simulink model "DR18E_Testpult"  (R2017a)
settings: Solver=ode1  StartTime=0.0  StopTime=Inf  FixedStep=0.001  RelTol=1e-3
PostLoadFcn:
  | , if any(exist('dsrtsu_mdlpostloadfcn', 'file') == [2, 3, 6]), try dsrtsu_mdlpostloadfcn('Execute', bdroot); catch fprintf('Error in PostLoadFcn (dsrtsu_mdlpostloadfcn) for model "%s":\n %s\n', bdroot, lasterr); end, end,
model workspace: external: MATLAB File C:\Users\DeltaRacing\Documents\dSPACE\MABX_DR18E\Model\DR18E_MABX_Parameter.m (data not in the file)
values from neighbouring files (symbols this model uses):
  am = 1/Ts    (= 1)    [DR18E_MABX_Parameter.m]
  bm = K/Ts    (= 0.05)    [DR18E_MABX_Parameter.m]
  cf = 41350    [DR18E_MABX_Parameter.m]
  cr = 41350    [DR18E_MABX_Parameter.m]
  Derating_HV_Battery_Kapa = 1    [DR18E_MABX_Parameter.m]
  Derating_Start_km = 16    [DR18E_MABX_Parameter.m]
  Drive_Mode = 0    [DR18E_MABX_Parameter.m]
  g = 1    [DR18E_MABX_Parameter.m]
  Gas_Modus = 2    [DR18E_MABX_Parameter.m]
  HV_Power_max = 80    [DR18E_MABX_Parameter.m]
  i_Getriebe = 3.3    [DR18E_MABX_Parameter.m]
  i_Lenkgetriebe = 4.32    [DR18E_MABX_Parameter.m]
  K_SET = 1    [DR18E_MABX_Parameter.m]
  Kapazitaet_HV_Battery_kWh = 6.6    [DR18E_MABX_Parameter.m]
  KW_T_Soll = 37    [DR18E_MABX_Parameter.m]
  lf = 1.2    [DR18E_MABX_Parameter.m]
  lr = 1.15    [DR18E_MABX_Parameter.m]
  m = 310    [DR18E_MABX_Parameter.m]
  M_max = 150    [DR18E_MABX_Parameter.m]
  Power_Limit_onoff = 0    [DR18E_MABX_Parameter.m]
  Reifenradius = 0.2351    [DR18E_MABX_Parameter.m]
  Strecke_Endu_km = 22    [DR18E_MABX_Parameter.m]
  TC_Decr_Gas = 0.00005    (= 5e-05)    [DR18E_MABX_Parameter.m]
  TC_Derivative = 0.4    [DR18E_MABX_Parameter.m]
  TC_Incr_Gas = 0.005    [DR18E_MABX_Parameter.m]
  TC_On = 0    [DR18E_MABX_Parameter.m]
  TC_Relay_Off = 0.065    [DR18E_MABX_Parameter.m]
  TC_Relay_On = 0.07    [DR18E_MABX_Parameter.m]
  TV_Mode = 2    [DR18E_MABX_Parameter.m]
  TV_On = 0    [DR18E_MABX_Parameter.m]
  TV_Override = 1    [DR18E_MABX_Parameter.m]
  y = 0.8    [DR18E_MABX_Parameter.m]
undefined symbols (not defined in the file or in its folder): D, DiscIntNeverNeededParam, I, K_OL, P
libraries: simulink x288, rtican x105, rtiusbflightreclib x40, rti1401lib_dio_type3 x10, simulink_extras x10, rti1401lib_adc_type4 x8, rti1401lib_II_base x7
(part 1 of 28)
Description:
  | Standard RTI1401 template.
  | Supported Matlab version:  R2017a.
settings Model: Tag=RTI1401  DSRTSU_INTERNAL_RTI_VER=500  DSRTSU_INTERNAL_RTI_TYPE=rti1401  DSRTSU_INTERNAL_RTIFPGA=90  Creator=DeltaRacing  LastModifiedBy=DeltaRacing
settings OptimizationCC: BlockReduction=off  OptimizeBlockIOStorage=off  BufferReuse=off  GlobalBufferReuse=off  ExpressionFolding=off  LocalBlockOutputs=off
settings DebuggingCC: SFNoUnconditionalDefaultTransitionDiag=warning
settings HardwareCC: ProdBitPerPointer=32  ProdBitPerSizeT=32  ProdBitPerPtrDiffT=32  ProdLargestAtomicInteger=Integer  ProdEndianess=BigEndian  ProdWordSize=32  ProdHWDeviceType=Custom Processor->Custom  TargetIntDivRoundTo=Zero  TargetEndianess=BigEndian  TargetHWDeviceType=Custom Processor->Custom
settings SFSimCC: MATLABDynamicMemAlloc=off
settings RTWCC: SystemTargetFile=rti1401.tlc  MakeCommand=make_rti  TemplateMakefile=rti1401.tmf  Description=dSPACE DS1401 Hardware Platform
settings RTWCC: CustomSource=|
  | flightrecsetup.c
  | DsFlRecUSB.c
settings STFCustomTargetCC: ParMdlRefBuildCompliant=on  GRTInterface=off  SystemTargetFile=rti1401.tlc
settings GRTTargetCC: TargetLangStandard=C89/C90 (ANSI)  CompOptLevelCompliant=off  ConcurrentExecutionCompliant=off  CombineOutputUpdateFcns=off  MatFileLogging=off  CPPClassGenCompliant=off  UseToolchainInfoCompliant=off
settings ConfigComp: CovMetricSettings=dswe

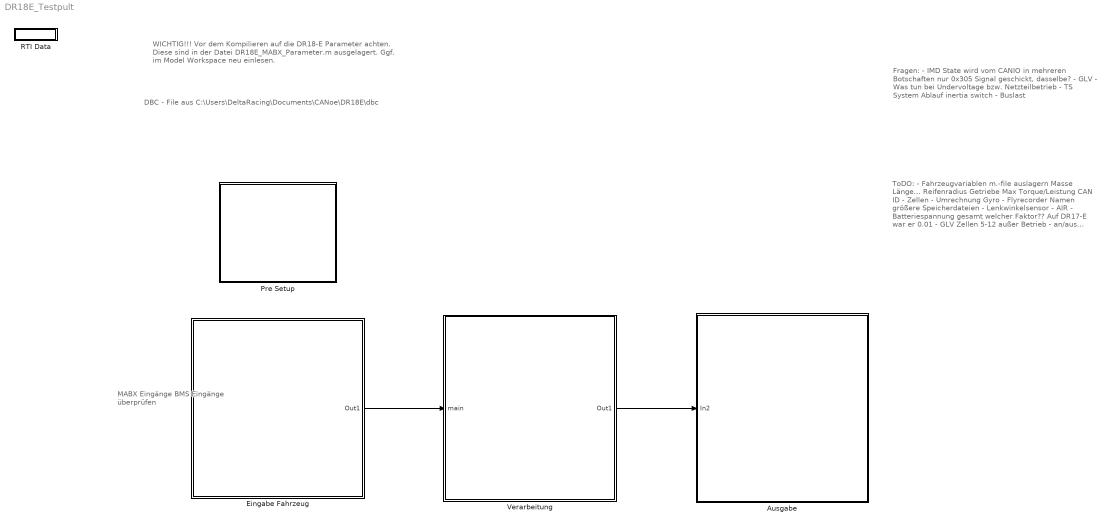
== system DR18E_Testpult ==
  note: WICHTIG!!!
      |
      | Vor dem Kompilieren auf die DR18-E Parameter achten.
      | Diese sind in der Datei DR18E_MABX_Parameter.m ausgelagert.
      | Ggf. im Model Workspace neu einlesen.
  note: MABX Eingänge
      | BMS Eingänge
      |
      | überprüfen
  note: DBC - File aus C:\Users\DeltaRacing\Documents\CANoe\DR18E\dbc
  note: Fragen:
      |
      | - IMD State wird vom CANIO in mehreren Botschaften
      | 		nur 0x305 Signal
      |  geschickt, dasselbe?
      | - GLV - Was tun bei Undervoltage bzw. Netzteilbetrieb
      | - TS System Ablauf
      | 	inertia switch
      | - Buslast
  note: ToDO:
      |
      | - Fahrzeugvariablen m.-file auslagern
      | 	Masse
      | 	Länge...
      | 	Reifenradius
      | 	Getriebe
      | 	Max Torque/Leistung
      | 	CAN ID - Zellen
      | - Umrechnung Gyro
      | - Flyrecorder
      | 	Namen
      | 	größere Speicherdateien
      | - Lenkwinkelsensor
      | - AIR
      | - Batteriespannung gesamt
      | 	welcher Faktor?? Auf DR17-E war er 0.01
      | - GLV Zellen 5-12 außer Betrieb
      | - an/aus Signale in dbc verankern (mal 255)
      | 	in dbc unsigned Variable und Faktor 255
      | - Sendezeiten in der dbc üperprüfen
      | 		Botschaft/Signal.. onchange cyclic
      | - TV Torque dazuaddieren Regel raussuchen
      | - BMS Generell
      | 		AMS Relay, 0x170, 0x231-2
      | - Unterschied zw. Speaker und Sound - State Machine
      | - Inverter Status Fehler Bit 31 überprüfen
      | - Skalierung Inverterwerte
      | 	Drehzahl Umrechung - 4000/2^15
      | 	Warum 4000?
      | - Rückwärtsgang
      | - BSPD Status - NOT OPERATOR? Warum
  Ausgabe : Subsystem
  Eingabe Fahrzeug : Subsystem
  Pre Setup : Subsystem
  RTI Data : Subsystem  Tag=struct('RTIDataServer',struct('RTIDataServerVs','2','RTIModelDescription','struct(''main'',''DR18E_Testpult'',''sub'','''',''isMp'',0)'))  LoadFcn="if exist('rtidc'), try,  rtidc('DataHostBlockClbLoad', gcbh); catch, disp(['Warning: ''LoadFcn'' for RTI Data block failed: ' lasterr]); end, end,"  mask(RTI_DATA_HOST){}
      mask help:
      | RTI Data Block.
      | This block is used by RTI to store internal model-dependent data.
      | Please keep this block on the root level of the model. Deleting this block will result in data loss.
      |
      | NEVER DELETE OR COPY THIS BLOCK!
      settings: CopyFcn="if exist('rtidc'), try,  rtidc('DataHostBlockClbCopy', gcbh); catch, disp(['Warning: ''CopyFcn'' for RTI Data block failed: ' lasterr]); end, end,"  DeleteFcn="if exist('rtidc'), try,  rtidc('DataHostBlockClbDelete', gcbh); catch, disp(['Warning: ''DeleteFcn'' for RTI Data block failed: ' lasterr]); end, end,"  ModelCloseFcn="if exist('rtidc'), try,  rtidc('DataHostBlockClbModelClose', gcbh); catch, disp(['Warning: ''ModelCloseFcn'' for RTI Data block failed: ' lasterr]); end, end,"  PreSaveFcn="if exist('rtidc'), try,  rtidc('DataHostBlockClbPreSave', gcbh); catch, disp(['Warning: ''PreSaveFcn'' for RTI Data block failed: ' lasterr]); end, end,"  PostSaveFcn="if exist('rtidc'), try,  rtidc('DataHostBlockClbPostSave', gcbh); catch, disp(['Warning: ''PostSaveFcn'' for RTI Data block failed: ' lasterr]); end, end,"  NameChangeFcn="if exist('rtidc'), try,  rtidc('DataHostBlockClbNameChange', gcbh); catch, disp(['Warning: ''NameChangeFcn'' for RTI Data block failed: ' lasterr]); end, end,"
      mask Help:
      | RTI Data Block.
      | This block is used by RTI to store internal model-dependent data.
      | Please keep this block on the root level of the model. Deleting this block will result in data loss.
      | 
      | NEVER DELETE OR COPY THIS BLOCK!
      mask Display:
      | text(0.5, 0.5, 'RTI Data', 'HorizontalAlignment', 'center');
      | plot([1 0]);
  Verarbeitung : Subsystem
  wires:
  Eingabe Fahrzeug/1(Out1) -> Verarbeitung/1(main)
  Verarbeitung/1(Out1) -> Ausgabe/1(In2)

== system DR18E_Testpult/Ausgabe ==
  In2 : Inport
  AMS : Subsystem
  Bus Selector : BusSelector  OutputSignals=Outputs_StateMachine.O_Inverter_TX_Mode,Outputs_StateMachine.UmrichterInit,Torque_L_R_Nm,Outputs_StateMachine.UniversalTX.RegID_L_R,Outputs_StateMachine.UniversalTX.Value32_L_R
  Bus Selector1 : BusSelector  OutputSignals=Outputs_StateMachine.O_Sicherheitskreis_Enable,Bremse_bin,Outputs_StateMachine.O_SpeakerEnable,PumpePWM,LüfterPWM,Outputs_StateMachine.O_Precharge_Enable,Outputs_StateMachine.O_InverterFRE
  Bus Selector2 : BusSelector  OutputSignals=Outputs_StateMachine.O_ErrorNr,Outputs_StateMachine.O_State,M_max,LED Bar Vektor.LED Bar Vektor
  Bus Selector3 : BusSelector  OutputSignals=Outputs_StateMachine.O_fBlink_Start,Sicherheitskreis,LV_Undervoltage
  Bus Selector4 : BusSelector  OutputSignals=A_AMS_out,A_IMD_out
  Bus Selector5 : BusSelector  OutputSignals=Lüfter HV Battery
  Bus Selector6 : BusSelector  OutputSignals=Bus_Input.Umrichter.U1.Mot_Temp,Bus_Input.Umrichter.U2.Mot_Temp,Bus_Input.Umrichter.U1.InverterTemp,Bus_Input.Umrichter.U2.InverterTemp
  CANIO : Subsystem
  Diagnose : Subsystem
  Display : Subsystem
  Inverter TX : Subsystem
  SensorboardMitte : Subsystem
  or : Logic  Operator=OR  AllPortsSameDT=off  OutDataTypeStr=boolean
  wires:
  In2/1 -> Bus Selector6/1, Bus Selector5/1, Bus Selector1/1, Bus Selector/1, Bus Selector3/1, Bus Selector2/1
  Bus Selector1/1 -> CANIO/1(Sicherheitskreis)  "<O_Sicherheitskreis_Enable>"
  Bus Selector1/3 -> CANIO/3(Speaker)  "<O_SpeakerEnable>"
  Bus Selector1/4 -> CANIO/4(Wasserpumpe)  "<PumpePWM>"
  Bus Selector1/5 -> CANIO/5(Lüfter)  "<LüfterPWM>"
  Bus Selector1/6 -> CANIO/6(Precharge)  "<O_Precharge_Enable>"
  Bus Selector1/7 -> CANIO/7(Inverter Enable)  "<O_InverterFRE>"
  Bus Selector/1 -> Inverter TX/1(Inverter_TX_Mode)  "<O_Inverter_TX_Mode>"
  Bus Selector/2 -> Inverter TX/2(Init_Values)  "<UmrichterInit>"
  Bus Selector/3 -> Inverter TX/3(Torque_L_R_Nm)  "<Torque_L_R_Nm>"
  Bus Selector/4 -> Inverter TX/4(RegID_L_R1)  "<RegID_L_R>"
  Bus Selector/5 -> Inverter TX/5(Values_L_R_32bit)  "<Value32_L_R>"
  Bus Selector2/1 -> Display/1(ErrorNo)  "<O_ErrorNr>"
  Bus Selector2/2 -> Display/2(State)  "<O_State>"
  Bus Selector3/1 -> SensorboardMitte/1(Starttaster)  "<O_fBlink_Start>"
  Bus Selector1/2 -> CANIO/2(Bremslicht)  "<Bremse_bin>"
  Bus Selector3/2 -> SensorboardMitte/2(DasboardNotausLed)  "<Sicherheitskreis>"
  [vec_Sicherheitskreis] -> Bus Selector4/1
  Bus Selector4/2 -> SensorboardMitte/4(DashboardIMDLed)  "<A_IMD_out>"
  Bus Selector3/3 -> or/1  "<LV_Undervoltage>"
  Bus Selector4/1 -> or/2  "<A_AMS_out>"
  or/1 -> SensorboardMitte/3("DashboardAMSLed ")
  Bus Selector5/1 -> AMS/1(Lüfter HV Battery)  "<Lüfter HV Battery>"
  Bus Selector2/3 -> Display/3("TorqueMax ")  "<M_max>"
  Bus Selector2/4 -> Display/4(LED Bar)  "<LED Bar Vektor>"
  Bus Selector6/1 -> Diagnose/1(Motor 1 Temperatur)  "<Mot_Temp>"
  Bus Selector6/2 -> Diagnose/2(Motor 2 Temperatur)  "<Mot_Temp>"
  Bus Selector6/3 -> Diagnose/3(IGBT 1 Temperatur)  "<InverterTemp>"
  Bus Selector6/4 -> Diagnose/4(IGBT 2 Temperatur)  "<InverterTemp>"

== system DR18E_Testpult/Eingabe Fahrzeug ==
  BMS : Subsystem
  Bus Creator : BusCreator  Inputs=11
  CAN IO : Subsystem
  "GLV AMS " : Subsystem
  Gyro : Subsystem
  Inverter Feedback Messages : Subsystem
  Lenkwinkelgeber : Subsystem
  MicroAutoBox : Subsystem
  Sensorboard Front : Subsystem
  Sensorboard Mitte : Subsystem
  Sensorboard Rear : Subsystem
  Out1 : Outport
  wires:
  Bus Creator/1 -> Out1/1
  Gyro/1(Gyro) -> Bus Creator/2
  Sensorboard Mitte/1(SensorboardMitteOut) -> Bus Creator/3
  Sensorboard Front/1(SensorboardFrontOut) -> Bus Creator/1
  MicroAutoBox/1(MicroAutoBox) -> Bus Creator/11
  Lenkwinkelgeber/1(LenkwinkelgeberOut) -> Bus Creator/5
  Inverter Feedback Messages/1(Out1) -> Bus Creator/6
  BMS/1(BMS Voltage) -> Bus Creator/7
  CAN IO/1(CANIOOut) -> Bus Creator/9
  Sensorboard Rear/1(SensorboardRearOut) -> Bus Creator/4
  "GLV AMS "/1(GLVAMSOut) -> Bus Creator/10
  BMS/2(Out2) -> Bus Creator/8

== system DR18E_Testpult/Pre Setup ==
  note: MABX ZIF Connector
      | CAN 3
  note: MABX ZIF Connector
      | CAN 1
  note: MABX ZIF Connector
      | CAN 2
  CAN 1 - Body : rtican/RTICAN CONTROLLER SETUP   Reserved1=[]  Reserved2=[]  Reserved3=[]  Reserved4=[]  AcceptanceMask=[]  ArbitrationField=[]  Parameters=[]  SFcnRTICANSettings=[]  MS_Struct=[]  BoardTypeNo=[]  BoardNo=[]  ChannelNo=[]  DialogFcn=[]  UnitName=[]  Revision=[]  UnitValues=[]  DSProperties=struct('RTI',struct('Version',uint32(12),'BlockType',struct('isSLSource',uint8(0),'isSLSink',uint8(0),'isHWSource',uint8(0),'isHWSink',uint8(0),'isSetup',uint8(1),'isInline',uint8(1),'isNonInline',uint8(0),'isInterrupt',uint8(0),'isChannelwise',uint8(0)),'IOBoardType','RTICAN','UnitType','NON_MESSAGE','Identifier','MASTER','DialogType','ML','BlockSet','RTICAN','SlaveProcessor','CAN'))  RTIBlockInterface=struct('InputPortsWidth',int32(0),'InputPortsActive',0,'OutputPortsWidth',int32(0),'OutputPortsActive',0,'DialogFcn','rtican_master_setup_gui','BlockDisplay',{{['CAN CONTROLLER\n SETUP'],'center'}},'IconTransparency','on','InitLevel',3,'IWork',{{{'',uint32(2)}}},'BlockName',struct('Token',{{'CAN_TYPE','_SETUP_M','_C'}},'BlockParam',{{'BoardTypeNo','BoardNo','ChannelNo'}}),'ParameterTunableNames',{{}})  RTIBlockParameters="struct('BoardTypeNo',{{1,'OFF',[]}},'BoardNo',{{2,'ON',[1 16]}},'ChannelNo',{{1,'ON',[1 2]}},'AcceptanceMask',{{0,'OFF',[]}},'ArbitrationField',{{0,'OFF',[]}},'Parameters',{{struct('Config',struct('Baudrate',500,'SampleMode',1,'UsedParamSet',1,'validSettings',1,'isBTRvalues',0,'Advanced',struct('Baudrate',{500,500,500},'Frequency',{24000000,36000000,64000000},'Settings',{struct('SMPL',0,'BRP',0,'NBT',24,'TSEG1',15,'TSEG2',6,'SJW',0,'SP',70),struct('SMPL',0,'BRP',1,'NBT',18,'TSEG1',11,'TSEG2',4,'SJW',0,'SP',72),struct('SMPL',0,'BRP',3,'NBT',16,'TSEG1',9,'TSEG2',4,'SJW',0,'SP',68)},'BTR0',{0,1,3},'BTR1',{111,75,73})),'configType',1,'Options',struct('DataFileSelected',1,'DataFileName',{{'..\\..\\..\\canoe\\dr18e_test\\dr18e\\dbc\\dr18e.dbc'}},'DataFileDate',{{['16-Feb-2019 13:23:09']}},'InterfaceFcn','rtican_dbc_file_parser','InterfaceFcnFileName','','LabelConfigType','volatile','AcceptanceMaskSelected',0,'MsgDataType','AllwaysDouble','NumType','hex','MaskType','STD','AcceptanceMask',0,'ArbitrationField',0,'UseMultipleMessageAccess',0),'RxReceiveStdOptions',struct('RxServiceStdEnabled',0,'RxServiceStdMsgIdent',1000,'RxServiceStdIdentNumType',1,'RxServiceStdIdentMask',0,'RxServiceStdMaskNumType',1,'RxServiceStdQueueSize',64),'RxReceiveXtdOptions',struct('RxServiceXtdEnabled',0,'RxServiceXtdMsgIdent',1001,'RxServiceXtdIdentNumType',1,'RxServiceXtdIdentMask',0,'RxServiceXtdMaskNumType',1,'RxServiceXtdQueueSize',64),'PartialNetworkingOptions',struct('switchedon',0,'format',1,'idmask',['    XXXXX XXXXXXXX XXXXXXXX XXXXXXXX'],'idcode','0','idfilter','0','datamaskused',0,'datalength',1,'datamask','0x0000000000000000','partialnetworkenable',0),'general',struct('Termination_common',1,'Termination_C252',1,'BusConfigurationRegister',0,'Transceiver','ISO11898','isFromLib',0)),'OFF',[]}},'CCPParameters',{{struct('CRO',struct('Format','STD','NumFormat','hex','Id',1639),'DTO',struct('Format','STD','NumFormat','hex','Id',2017),'StationAdr',struct('NumFormat','hex','Value',57),'StationId',struct('Value',['dSPACE CCP Service']),'Enabled',0),'OFF',[]}},'XCPParameters',{{struct('MASTER',struct('Format','STD','NumFormat','hex','Id',256),'SLAVE',struct('Format','STD','NumFormat','hex','Id',510),'Enabled',0,'PIDTransmissionEnabled',0),'OFF',[]}},'GroupId',{{struct('Group',{{'RTICAN'}},'No',1,'Behavior',{{'EVER'}},'BlockType',{{'SOURCE'}},'NameChangeFlag',1),'OFF',[]}},'SFcnRTICANSettings',{{struct('Baudrate',500,'configType',1,'AdvancedConfig',struct('Frequency',{},'BTR0',{},'BTR1',{}),'UsedParamSet',1,'STDMaskSelected','no','XTDMaskSelected','no','BoardType','DS1','BoardNo',2,'ControllerNo',1,'Transceiver','ISO11898','BusConfigRegister',0,'TerminationRes',120,'UseMultipleMessageAccess','no','STDRXSrvcUsed','no','STDRXSrvcMsgId',1000,'STDRXSrvcMsgMask',0,'STDRXSrvcQueueSize',64,'XTDRXSrvcUsed','no','XTDRXSrvcMsgId',1001,'XTDRXSrvcQueueSize',64,'XTDRXSrvcMsgMask',0,'PN_IsPNTransciever',0,'PN_IsPNEnabled',0,'PN_MsgFormat',1,'PN_idcode',0,'PN_idmask',2047,'PN_datamaskused',0,'PN_datalength',0,'PN_datamask',['0xFF, 0xFF, 0xFF, 0xFF, 0xFF, 0xFF, 0xFF, 0xFF']),'OFF',[]}},'SFcnRTICCPSettings',{{struct('CRO',struct('Format','STD','NumFormat','hex','Id',1639),'DTO',struct('Format','STD','NumFormat','hex','Id',2017),'StationAdr',struct('NumFormat','hex','Value',57),'StationId',struct('Value',['dSPACE CCP Service']),'Enabled',0),'OFF',[]}},'SFcnRTIXCPSettings',{{struct('MASTER',struct('Format','STD','NumFormat','hex','Id',256),'SLAVE',struct('Format','STD','NumFormat','hex','Id',510),'Enabled',0,'PIDTransmissionEnabled',0),'OFF',[]}},'TLCFileName',{{'rtican_master_setup','OFF',[]}})"  RTISFcnParameters=struct('SFcnRTICANSettings','struct','SFcnRTICCPSettings','struct','SFcnRTIXCPSettings','struct','AcceptanceMask','int32','ArbitrationField','int32','TLCFileName','char')  RTIBlockParaDefault="struct('BoardTypeNo',4302,'BoardNo',1,'ChannelNo',1,'AcceptanceMask',0,'ArbitrationField',0,'Parameters',struct('Config',struct('Baudrate',500,'SampleMode',1,'UsedParamSet',1,'validSettings',1,'isBTRvalues',0,'Advanced',struct('Frequency',16000000,'BTR0',64,'BTR1',28,'Settings',struct('SMPL',0,'BRP',0,'NBT',16,'TSEG1',12,'TSEG2',1,'SJW',1,'SP',87))),'configType',1,'Options',struct('DataFileSelected',0,'DataFileName',{{['<no datafile support>']}},'DataFileDate',{{''}},'InterfaceFcn','rtican_dbc_file_parser','InterfaceFcnFileName','','LabelConfigType','volatile','AcceptanceMaskSelected',0,'MsgDataType','AllwaysDouble','NumType','hex','MaskType','STD','AcceptanceMask',0,'ArbitrationField',0,'UseMultipleMessageAccess',0),'RxReceiveStdOptions',struct('RxServiceStdEnabled',0,'RxServiceStdMsgIdent',1000,'RxServiceStdIdentNumType',1,'RxServiceStdIdentMask',0,'RxServiceStdMaskNumType',1,'RxServiceStdQueueSize',64),'RxReceiveXtdOptions',struct('RxServiceXtdEnabled',0,'RxServiceXtdMsgIdent',1001,'RxServiceXtdIdentNumType',1,'RxServiceXtdIdentMask',0,'RxServiceXtdMaskNumType',1,'RxServiceXtdQueueSize',64),'PartialNetworkingOptions',struct('switchedon',0,'format',1,'idmask',['    XXXXX XXXXXXXX XXXXXXXX XXXXXXXX'],'idcode','0','idfilter','0','datamaskused',0,'datalength',1,'datamask','0x0000000000000000','partialnetworkenable',0),'general',struct('Termination_common',1,'Termination_C252',1,'BusConfigurationRegister',0,'Transceiver','ISO11898','isFromLib',1)),'CCPParameters',struct('CRO',struct('Format','STD','NumFormat','hex','Id',1639),'DTO',struct('Format','STD','NumFormat','hex','Id',2017),'StationAdr',struct('NumFormat','hex','Value',57),'StationId',struct('Value',['dSPACE CCP Service']),'Enabled',0),'XCPParameters',struct('MASTER',struct('Format','STD','NumFormat','hex','Id',256),'SLAVE',struct('Format','STD','NumFormat','hex','Id',510),'Enabled',0,'PIDTransmissionEnabled',0),'GroupId',struct('Group',{{'RTICAN'}},'No',1,'Behavior',{{'EVER'}},'BlockType',{{'SOURCE'}},'NameChangeFlag',1),'SFcnRTICANSettings',struct('Baudrate',500,'configType',1,'AdvandedConfig',struct('Frequency',16000000,'BTR0','0x40','BTR1','0x1C'),'UsedParamSet',1,'STDMaskSelected','no','XTDMaskSelected','no','BoardType','DS4302','BoardNo',1,'ControllerNo',1,'Transceiver','ISO11898','BusConfigRegister',0,'TerminationRes',120,'UseMultipleMessageAccess','no','STDRXSrvcUsed','no','STDRXSrvcMsgId',1000,'STDRXSrvcMsgMask',0,'STDRXSrvcQueueSize',64,'XTDRXSrvcUsed','no','XTDRXSrvcMsgId',1001,'XTDRXSrvcQueueSize',64,'XTDRXSrvcMsgMask',0),'SFcnRTICCPSettings',struct('CRO',struct('Format','STD','NumFormat','hex','Id',1639),'DTO',struct('Format','STD','NumFormat','hex','Id',2017),'StationAdr',struct('NumFormat','hex','Value',57),'StationId',struct('Value',['dSPACE CCP Service']),'Enabled',0),'SFcnRTIXCPSettings',struct('MASTER',struct('Format','STD','NumFormat','hex','Id',256),'SLAVE',struct('Format','STD','NumFormat','hex','Id',510),'Enabled',0,'PIDTransmissionEnabled',0),'TLCFileName','rtican_master_setup')"
      settings: AttributesFormatString=Group Id: RTICAN1\n  SourceProductName=dSPACE RTI CAN Blockset
  CAN 1 Recovery : Constant  Value=0
  CAN1 Status : rtican/RTICAN Status   Reserved1=[]  Reserved2=[]  Reserved3=[]  Reserved4=[]  DialogFcn=[]  UnitName=[]  SFcnRTICANStatus=[]  BoardTypeNo=[]  BoardNo=[]  ChannelNo=[]  Parameters=[]  Revision=[]  UnitValues=[]  DSProperties=struct('RTI',struct('Version',uint32(4),'BlockType',struct('isSLSource',uint8(1),'isSLSink',uint8(0),'isHWSource',uint8(0),'isHWSink',uint8(0),'isSetup',uint8(0),'isInline',uint8(1),'isNonInline',uint8(0),'isInterrupt',uint8(0),'isChannelwise',uint8(0)),'IOBoardType','RTICAN','UnitType','NON_MESSAGE','Identifier','STATUS','DialogType','ML','BlockSet','RTICAN','SlaveProcessor','CAN'))  RTIBlockInterface=struct('OutputPortsWidth',int32([1 1 1 1 1 1 1 1 1 1 1 1]),'OutputPortsActive',[1 1 1 1 1 1 1 1 1 1 0 0],'OutputPortsName',{{'Status',['Stuff errors'],['Format errors'],['Ack errors'],['Bit 0 errors'],['Bit 1 errors'],['CRC errors'],['RX lost'],['RX ok'],['TX ok'],['FT Status'],['FT error count']}},'OutputPortsDataType',{{'SS_UINT32','SS_UINT32','SS_UINT32','SS_UINT32','SS_UINT32','SS_UINT32','SS_UINT32','SS_UINT32','SS_UINT32','SS_UINT32','SS_UINT32','SS_UINT32'}},'DialogFcn','rtican_status_gui','BlockDisplay',{{'','center'}},'IconTransparency','on','ParameterTunableNames',{{}},'InitLevel',3,'BlockName',struct('Token',{{'CAN_TYPE','_STATUS_M','_C'}},'BlockParam',{{'BoardTypeNo','BoardNo','ChannelNo'}}),'SampleTime',{{2^-1}})  RTIBlockParameters=struct('BoardTypeNo',{{1,'OFF',[]}},'BoardNo',{{2,'ON',[1 16]}},'ChannelNo',{{1,'ON',[1 2]}},'Parameters',{{struct('general',struct('isFromLib',0,'StatusFlags',{{1;1;1;1;1;1;1;1;1;1;0;0}}),'options',struct('SampleTime',2^-1)),'OFF',[]}},'GroupId',{{struct('Group','RTICAN','No',1,'Behavior','NAMECHANGE','BlockType','SINK','NameChangeFlag',0),'OFF',[]}},'SFcnRTICANStatus',{{struct('Output',struct('Name',{'Status','StuffErrors','FormatErrors','AckErrors','Bit0Errors','Bit1Errors','CRCErrors','RXLost','RXOK','TXOK','FTStatus','FTErrorCount'},'Selected',{'yes','yes','yes','yes','yes','yes','yes','yes','yes','yes','no','no'}),'ControllerNo',1,'BoardNo',2,'BoardType','DS1','PortDatatype','UInt32'),'OFF',[]}},'TLCFileName',{{'rtican_status','OFF',[]}})  RTISFcnParameters=struct('SFcnRTICANStatus','struct','TLCFileName','char')  RTIBlockParaDefault=struct('BoardTypeNo',4302,'BoardNo',1,'ChannelNo',1,'Parameters',struct('general',struct('StatusFlags',{{1;1;1;1;1;1;1;1;1;1;0;0}},'isFromLib',1),'options',struct('SampleTime',2^-1)),'GroupId',struct('Group',{{'RTICAN'}},'No',1,'Behavior',{{'NAMECHANGE'}},'BlockType',{{'SINK'}},'NameChangeFlag',0),'SFcnRTICANStatus',struct('Output',struct('Name',{'Status','StuffErrors','FormatErrors','AckErrors','Bit0Errors','Bit1Errors','CRCErrors','RXLost','RXOK','TXOK','FTStatus','FTErrorCount'},'Selected',{'yes','yes','yes','yes','yes','yes','yes','yes','yes','yes','no','no'}),'ControllerNo',1,'BoardNo',1,'BoardType','DS4302','PortDatatype','real_T'),'TLCFileName','rtican_status')
      settings: AttributesFormatString=Group Id: RTICAN1\n  SourceProductName=dSPACE RTI CAN Blockset
  CAN2 - Inv 1 links : rtican/RTICAN CONTROLLER SETUP   Reserved1=[]  Reserved2=[]  Reserved3=[]  Reserved4=[]  AcceptanceMask=[]  ArbitrationField=[]  Parameters=[]  SFcnRTICANSettings=[]  MS_Struct=[]  BoardTypeNo=[]  BoardNo=[]  ChannelNo=[]  DialogFcn=[]  UnitName=[]  Revision=[]  UnitValues=[]  DSProperties=struct('RTI',struct('Version',uint32(12),'BlockType',struct('isSLSource',uint8(0),'isSLSink',uint8(0),'isHWSource',uint8(0),'isHWSink',uint8(0),'isSetup',uint8(1),'isInline',uint8(1),'isNonInline',uint8(0),'isInterrupt',uint8(0),'isChannelwise',uint8(0)),'IOBoardType','RTICAN','UnitType','NON_MESSAGE','Identifier','MASTER','DialogType','ML','BlockSet','RTICAN','SlaveProcessor','CAN'))  RTIBlockInterface=struct('InputPortsWidth',int32(0),'InputPortsActive',0,'OutputPortsWidth',int32(0),'OutputPortsActive',0,'DialogFcn','rtican_master_setup_gui','BlockDisplay',{{['CAN CONTROLLER\n SETUP'],'center'}},'IconTransparency','on','InitLevel',3,'IWork',{{{'',uint32(2)}}},'BlockName',struct('Token',{{'CAN_TYPE','_SETUP_M','_C'}},'BlockParam',{{'BoardTypeNo','BoardNo','ChannelNo'}}),'ParameterTunableNames',{{}})  RTIBlockParameters="struct('BoardTypeNo',{{1,'OFF',[]}},'BoardNo',{{1,'ON',[1 16]}},'ChannelNo',{{1,'ON',[1 2]}},'AcceptanceMask',{{0,'OFF',[]}},'ArbitrationField',{{0,'OFF',[]}},'Parameters',{{struct('Config',struct('Baudrate',500,'SampleMode',1,'UsedParamSet',1,'validSettings',1,'isBTRvalues',0,'Advanced',struct('Baudrate',{500,500,500},'Frequency',{24000000,36000000,64000000},'Settings',{struct('SMPL',0,'BRP',0,'NBT',24,'TSEG1',15,'TSEG2',6,'SJW',3,'SP',70),struct('SMPL',0,'BRP',1,'NBT',18,'TSEG1',14,'TSEG2',1,'SJW',1,'SP',88),struct('SMPL',0,'BRP',3,'NBT',16,'TSEG1',12,'TSEG2',1,'SJW',1,'SP',87)},'BTR0',{192,65,67},'BTR1',{111,30,28})),'configType',1,'Options',struct('DataFileSelected',0,'DataFileName',{{['<no datafile support>']}},'DataFileDate',{{''}},'InterfaceFcn','rtican_dbc_file_parser','InterfaceFcnFileName','','LabelConfigType','volatile','AcceptanceMaskSelected',0,'MsgDataType','AllwaysDouble','NumType','hex','MaskType','STD','AcceptanceMask',0,'ArbitrationField',0,'UseMultipleMessageAccess',1),'RxReceiveStdOptions',struct('RxServiceStdEnabled',0,'RxServiceStdMsgIdent',1000,'RxServiceStdIdentNumType',1,'RxServiceStdIdentMask',0,'RxServiceStdMaskNumType',1,'RxServiceStdQueueSize',64),'RxReceiveXtdOptions',struct('RxServiceXtdEnabled',0,'RxServiceXtdMsgIdent',1001,'RxServiceXtdIdentNumType',1,'RxServiceXtdIdentMask',0,'RxServiceXtdMaskNumType',1,'RxServiceXtdQueueSize',64),'PartialNetworkingOptions',struct('switchedon',0,'format',1,'idmask',['    XXXXX XXXXXXXX XXXXXXXX XXXXXXXX'],'idcode','0','idfilter','0','datamaskused',0,'datalength',1,'datamask','0x0000000000000000','partialnetworkenable',0),'general',struct('Termination_common',2,'Termination_C252',1,'BusConfigurationRegister',0,'Transceiver','ISO11898','isFromLib',0)),'OFF',[]}},'CCPParameters',{{struct('CRO',struct('Format','STD','NumFormat','hex','Id',1639),'DTO',struct('Format','STD','NumFormat','hex','Id',2017),'StationAdr',struct('NumFormat','hex','Value',57),'StationId',struct('Value',['dSPACE CCP Service']),'Enabled',0),'OFF',[]}},'XCPParameters',{{struct('MASTER',struct('Format','STD','NumFormat','hex','Id',256),'SLAVE',struct('Format','STD','NumFormat','hex','Id',510),'Enabled',0,'PIDTransmissionEnabled',0),'OFF',[]}},'GroupId',{{struct('Group',{{'RTICAN'}},'No',2,'Behavior',{{'EVER'}},'BlockType',{{'SOURCE'}},'NameChangeFlag',1),'OFF',[]}},'SFcnRTICANSettings',{{struct('Baudrate',500,'configType',1,'AdvancedConfig',struct('Frequency',{},'BTR0',{},'BTR1',{}),'UsedParamSet',1,'STDMaskSelected','no','XTDMaskSelected','no','BoardType','DS1','BoardNo',1,'ControllerNo',1,'Transceiver','ISO11898','BusConfigRegister',0,'TerminationRes',-1,'UseMultipleMessageAccess','yes','STDRXSrvcUsed','no','STDRXSrvcMsgId',1000,'STDRXSrvcMsgMask',0,'STDRXSrvcQueueSize',64,'XTDRXSrvcUsed','no','XTDRXSrvcMsgId',1001,'XTDRXSrvcQueueSize',64,'XTDRXSrvcMsgMask',0,'PN_IsPNTransciever',0,'PN_IsPNEnabled',0,'PN_MsgFormat',1,'PN_idcode',0,'PN_idmask',2047,'PN_datamaskused',0,'PN_datalength',0,'PN_datamask',['0xFF, 0xFF, 0xFF, 0xFF, 0xFF, 0xFF, 0xFF, 0xFF']),'OFF',[]}},'SFcnRTICCPSettings',{{struct('CRO',struct('Format','STD','NumFormat','hex','Id',1639),'DTO',struct('Format','STD','NumFormat','hex','Id',2017),'StationAdr',struct('NumFormat','hex','Value',57),'StationId',struct('Value',['dSPACE CCP Service']),'Enabled',0),'OFF',[]}},'SFcnRTIXCPSettings',{{struct('MASTER',struct('Format','STD','NumFormat','hex','Id',256),'SLAVE',struct('Format','STD','NumFormat','hex','Id',510),'Enabled',0,'PIDTransmissionEnabled',0),'OFF',[]}},'TLCFileName',{{'rtican_master_setup','OFF',[]}})"  RTISFcnParameters=struct('SFcnRTICANSettings','struct','SFcnRTICCPSettings','struct','SFcnRTIXCPSettings','struct','AcceptanceMask','int32','ArbitrationField','int32','TLCFileName','char')  RTIBlockParaDefault="struct('BoardTypeNo',4302,'BoardNo',1,'ChannelNo',1,'AcceptanceMask',0,'ArbitrationField',0,'Parameters',struct('Config',struct('Baudrate',500,'SampleMode',1,'UsedParamSet',1,'validSettings',1,'isBTRvalues',0,'Advanced',struct('Frequency',16000000,'BTR0',64,'BTR1',28,'Settings',struct('SMPL',0,'BRP',0,'NBT',16,'TSEG1',12,'TSEG2',1,'SJW',1,'SP',87))),'configType',1,'Options',struct('DataFileSelected',0,'DataFileName',{{['<no datafile support>']}},'DataFileDate',{{''}},'InterfaceFcn','rtican_dbc_file_parser','InterfaceFcnFileName','','LabelConfigType','volatile','AcceptanceMaskSelected',0,'MsgDataType','AllwaysDouble','NumType','hex','MaskType','STD','AcceptanceMask',0,'ArbitrationField',0,'UseMultipleMessageAccess',0),'RxReceiveStdOptions',struct('RxServiceStdEnabled',0,'RxServiceStdMsgIdent',1000,'RxServiceStdIdentNumType',1,'RxServiceStdIdentMask',0,'RxServiceStdMaskNumType',1,'RxServiceStdQueueSize',64),'RxReceiveXtdOptions',struct('RxServiceXtdEnabled',0,'RxServiceXtdMsgIdent',1001,'RxServiceXtdIdentNumType',1,'RxServiceXtdIdentMask',0,'RxServiceXtdMaskNumType',1,'RxServiceXtdQueueSize',64),'PartialNetworkingOptions',struct('switchedon',0,'format',1,'idmask',['    XXXXX XXXXXXXX XXXXXXXX XXXXXXXX'],'idcode','0','idfilter','0','datamaskused',0,'datalength',1,'datamask','0x0000000000000000','partialnetworkenable',0),'general',struct('Termination_common',1,'Termination_C252',1,'BusConfigurationRegister',0,'Transceiver','ISO11898','isFromLib',1)),'CCPParameters',struct('CRO',struct('Format','STD','NumFormat','hex','Id',1639),'DTO',struct('Format','STD','NumFormat','hex','Id',2017),'StationAdr',struct('NumFormat','hex','Value',57),'StationId',struct('Value',['dSPACE CCP Service']),'Enabled',0),'XCPParameters',struct('MASTER',struct('Format','STD','NumFormat','hex','Id',256),'SLAVE',struct('Format','STD','NumFormat','hex','Id',510),'Enabled',0,'PIDTransmissionEnabled',0),'GroupId',struct('Group',{{'RTICAN'}},'No',1,'Behavior',{{'EVER'}},'BlockType',{{'SOURCE'}},'NameChangeFlag',1),'SFcnRTICANSettings',struct('Baudrate',500,'configType',1,'AdvandedConfig',struct('Frequency',16000000,'BTR0','0x40','BTR1','0x1C'),'UsedParamSet',1,'STDMaskSelected','no','XTDMaskSelected','no','BoardType','DS4302','BoardNo',1,'ControllerNo',1,'Transceiver','ISO11898','BusConfigRegister',0,'TerminationRes',120,'UseMultipleMessageAccess','no','STDRXSrvcUsed','no','STDRXSrvcMsgId',1000,'STDRXSrvcMsgMask',0,'STDRXSrvcQueueSize',64,'XTDRXSrvcUsed','no','XTDRXSrvcMsgId',1001,'XTDRXSrvcQueueSize',64,'XTDRXSrvcMsgMask',0),'SFcnRTICCPSettings',struct('CRO',struct('Format','STD','NumFormat','hex','Id',1639),'DTO',struct('Format','STD','NumFormat','hex','Id',2017),'StationAdr',struct('NumFormat','hex','Value',57),'StationId',struct('Value',['dSPACE CCP Service']),'Enabled',0),'SFcnRTIXCPSettings',struct('MASTER',struct('Format','STD','NumFormat','hex','Id',256),'SLAVE',struct('Format','STD','NumFormat','hex','Id',510),'Enabled',0,'PIDTransmissionEnabled',0),'TLCFileName','rtican_master_setup')"
      settings: AttributesFormatString=Group Id: RTICAN2\n  SourceProductName=dSPACE RTI CAN Blockset
  CAN2 Status : rtican/RTICAN Status   Reserved1=[]  Reserved2=[]  Reserved3=[]  Reserved4=[]  DialogFcn=[]  UnitName=[]  SFcnRTICANStatus=[]  BoardTypeNo=[]  BoardNo=[]  ChannelNo=[]  Parameters=[]  Revision=[]  UnitValues=[]  DSProperties=struct('RTI',struct('Version',uint32(4),'BlockType',struct('isSLSource',uint8(1),'isSLSink',uint8(0),'isHWSource',uint8(0),'isHWSink',uint8(0),'isSetup',uint8(0),'isInline',uint8(1),'isNonInline',uint8(0),'isInterrupt',uint8(0),'isChannelwise',uint8(0)),'IOBoardType','RTICAN','UnitType','NON_MESSAGE','Identifier','STATUS','DialogType','ML','BlockSet','RTICAN','SlaveProcessor','CAN'))  RTIBlockInterface=struct('OutputPortsWidth',int32([1 1 1 1 1 1 1 1 1 1 1 1]),'OutputPortsActive',[1 1 1 1 1 1 1 1 1 1 0 0],'OutputPortsName',{{'Status',['Stuff errors'],['Format errors'],['Ack errors'],['Bit 0 errors'],['Bit 1 errors'],['CRC errors'],['RX lost'],['RX ok'],['TX ok'],['FT Status'],['FT error count']}},'OutputPortsDataType',{{'SS_UINT32','SS_UINT32','SS_UINT32','SS_UINT32','SS_UINT32','SS_UINT32','SS_UINT32','SS_UINT32','SS_UINT32','SS_UINT32','SS_UINT32','SS_UINT32'}},'DialogFcn','rtican_status_gui','BlockDisplay',{{'','center'}},'IconTransparency','on','ParameterTunableNames',{{}},'InitLevel',3,'BlockName',struct('Token',{{'CAN_TYPE','_STATUS_M','_C'}},'BlockParam',{{'BoardTypeNo','BoardNo','ChannelNo'}}),'SampleTime',{{2^-1}})  RTIBlockParameters=struct('BoardTypeNo',{{1,'OFF',[]}},'BoardNo',{{1,'ON',[1 16]}},'ChannelNo',{{1,'ON',[1 2]}},'Parameters',{{struct('general',struct('isFromLib',0,'StatusFlags',{{1;1;1;1;1;1;1;1;1;1;0;0}}),'options',struct('SampleTime',2^-1)),'OFF',[]}},'GroupId',{{struct('Group','RTICAN','No',2,'Behavior','NAMECHANGE','BlockType','SINK','NameChangeFlag',0),'OFF',[]}},'SFcnRTICANStatus',{{struct('Output',struct('Name',{'Status','StuffErrors','FormatErrors','AckErrors','Bit0Errors','Bit1Errors','CRCErrors','RXLost','RXOK','TXOK','FTStatus','FTErrorCount'},'Selected',{'yes','yes','yes','yes','yes','yes','yes','yes','yes','yes','no','no'}),'ControllerNo',1,'BoardNo',1,'BoardType','DS1','PortDatatype','UInt32'),'OFF',[]}},'TLCFileName',{{'rtican_status','OFF',[]}})  RTISFcnParameters=struct('SFcnRTICANStatus','struct','TLCFileName','char')  RTIBlockParaDefault=struct('BoardTypeNo',4302,'BoardNo',1,'ChannelNo',1,'Parameters',struct('general',struct('StatusFlags',{{1;1;1;1;1;1;1;1;1;1;0;0}},'isFromLib',1),'options',struct('SampleTime',2^-1)),'GroupId',struct('Group',{{'RTICAN'}},'No',1,'Behavior',{{'NAMECHANGE'}},'BlockType',{{'SINK'}},'NameChangeFlag',0),'SFcnRTICANStatus',struct('Output',struct('Name',{'Status','StuffErrors','FormatErrors','AckErrors','Bit0Errors','Bit1Errors','CRCErrors','RXLost','RXOK','TXOK','FTStatus','FTErrorCount'},'Selected',{'yes','yes','yes','yes','yes','yes','yes','yes','yes','yes','no','no'}),'ControllerNo',1,'BoardNo',1,'BoardType','DS4302','PortDatatype','real_T'),'TLCFileName','rtican_status')
      settings: AttributesFormatString=Group Id: RTICAN2\n  SourceProductName=dSPACE RTI CAN Blockset
  CAN3 - Inv 2 rechts : rtican/RTICAN CONTROLLER SETUP   Reserved1=[]  Reserved2=[]  Reserved3=[]  Reserved4=[]  AcceptanceMask=[]  ArbitrationField=[]  Parameters=[]  SFcnRTICANSettings=[]  MS_Struct=[]  BoardTypeNo=[]  BoardNo=[]  ChannelNo=[]  DialogFcn=[]  UnitName=[]  Revision=[]  UnitValues=[]  DSProperties=struct('RTI',struct('Version',uint32(12),'BlockType',struct('isSLSource',uint8(0),'isSLSink',uint8(0),'isHWSource',uint8(0),'isHWSink',uint8(0),'isSetup',uint8(1),'isInline',uint8(1),'isNonInline',uint8(0),'isInterrupt',uint8(0),'isChannelwise',uint8(0)),'IOBoardType','RTICAN','UnitType','NON_MESSAGE','Identifier','MASTER','DialogType','ML','BlockSet','RTICAN','SlaveProcessor','CAN'))  RTIBlockInterface=struct('InputPortsWidth',int32(0),'InputPortsActive',0,'OutputPortsWidth',int32(0),'OutputPortsActive',0,'DialogFcn','rtican_master_setup_gui','BlockDisplay',{{['CAN CONTROLLER\n SETUP'],'center'}},'IconTransparency','on','InitLevel',3,'IWork',{{{'',uint32(2)}}},'BlockName',struct('Token',{{'CAN_TYPE','_SETUP_M','_C'}},'BlockParam',{{'BoardTypeNo','BoardNo','ChannelNo'}}),'ParameterTunableNames',{{}})  RTIBlockParameters="struct('BoardTypeNo',{{1,'OFF',[]}},'BoardNo',{{1,'ON',[1 16]}},'ChannelNo',{{2,'ON',[1 2]}},'AcceptanceMask',{{0,'OFF',[]}},'ArbitrationField',{{0,'OFF',[]}},'Parameters',{{struct('Config',struct('Baudrate',500,'SampleMode',1,'UsedParamSet',1,'validSettings',1,'isBTRvalues',0,'Advanced',struct('Baudrate',{500,500,500},'Frequency',{24000000,36000000,64000000},'Settings',{struct('SMPL',0,'BRP',0,'NBT',24,'TSEG1',15,'TSEG2',6,'SJW',3,'SP',70),struct('SMPL',0,'BRP',1,'NBT',18,'TSEG1',14,'TSEG2',1,'SJW',1,'SP',88),struct('SMPL',0,'BRP',3,'NBT',16,'TSEG1',12,'TSEG2',1,'SJW',1,'SP',87)},'BTR0',{192,65,67},'BTR1',{111,30,28})),'configType',1,'Options',struct('DataFileSelected',0,'DataFileName',{{['<no datafile support>']}},'DataFileDate',{{''}},'InterfaceFcn','rtican_dbc_file_parser','InterfaceFcnFileName','','LabelConfigType','volatile','AcceptanceMaskSelected',0,'MsgDataType','AllwaysDouble','NumType','hex','MaskType','STD','AcceptanceMask',0,'ArbitrationField',0,'UseMultipleMessageAccess',1),'RxReceiveStdOptions',struct('RxServiceStdEnabled',0,'RxServiceStdMsgIdent',1000,'RxServiceStdIdentNumType',1,'RxServiceStdIdentMask',0,'RxServiceStdMaskNumType',1,'RxServiceStdQueueSize',64),'RxReceiveXtdOptions',struct('RxServiceXtdEnabled',0,'RxServiceXtdMsgIdent',1001,'RxServiceXtdIdentNumType',1,'RxServiceXtdIdentMask',0,'RxServiceXtdMaskNumType',1,'RxServiceXtdQueueSize',64),'PartialNetworkingOptions',struct('switchedon',0,'format',1,'idmask',['    XXXXX XXXXXXXX XXXXXXXX XXXXXXXX'],'idcode','0','idfilter','0','datamaskused',0,'datalength',1,'datamask','0x0000000000000000','partialnetworkenable',0),'general',struct('Termination_common',2,'Termination_C252',1,'BusConfigurationRegister',0,'Transceiver','ISO11898','isFromLib',0)),'OFF',[]}},'CCPParameters',{{struct('CRO',struct('Format','STD','NumFormat','hex','Id',1639),'DTO',struct('Format','STD','NumFormat','hex','Id',2017),'StationAdr',struct('NumFormat','hex','Value',57),'StationId',struct('Value',['dSPACE CCP Service']),'Enabled',0),'OFF',[]}},'XCPParameters',{{struct('MASTER',struct('Format','STD','NumFormat','hex','Id',256),'SLAVE',struct('Format','STD','NumFormat','hex','Id',510),'Enabled',0,'PIDTransmissionEnabled',0),'OFF',[]}},'GroupId',{{struct('Group',{{'RTICAN'}},'No',3,'Behavior',{{'EVER'}},'BlockType',{{'SOURCE'}},'NameChangeFlag',1),'OFF',[]}},'SFcnRTICANSettings',{{struct('Baudrate',500,'configType',1,'AdvancedConfig',struct('Frequency',{},'BTR0',{},'BTR1',{}),'UsedParamSet',1,'STDMaskSelected','no','XTDMaskSelected','no','BoardType','DS1','BoardNo',1,'ControllerNo',2,'Transceiver','ISO11898','BusConfigRegister',0,'TerminationRes',-1,'UseMultipleMessageAccess','yes','STDRXSrvcUsed','no','STDRXSrvcMsgId',1000,'STDRXSrvcMsgMask',0,'STDRXSrvcQueueSize',64,'XTDRXSrvcUsed','no','XTDRXSrvcMsgId',1001,'XTDRXSrvcQueueSize',64,'XTDRXSrvcMsgMask',0,'PN_IsPNTransciever',0,'PN_IsPNEnabled',0,'PN_MsgFormat',1,'PN_idcode',0,'PN_idmask',2047,'PN_datamaskused',0,'PN_datalength',0,'PN_datamask',['0xFF, 0xFF, 0xFF, 0xFF, 0xFF, 0xFF, 0xFF, 0xFF']),'OFF',[]}},'SFcnRTICCPSettings',{{struct('CRO',struct('Format','STD','NumFormat','hex','Id',1639),'DTO',struct('Format','STD','NumFormat','hex','Id',2017),'StationAdr',struct('NumFormat','hex','Value',57),'StationId',struct('Value',['dSPACE CCP Service']),'Enabled',0),'OFF',[]}},'SFcnRTIXCPSettings',{{struct('MASTER',struct('Format','STD','NumFormat','hex','Id',256),'SLAVE',struct('Format','STD','NumFormat','hex','Id',510),'Enabled',0,'PIDTransmissionEnabled',0),'OFF',[]}},'TLCFileName',{{'rtican_master_setup','OFF',[]}})"  RTISFcnParameters=struct('SFcnRTICANSettings','struct','SFcnRTICCPSettings','struct','SFcnRTIXCPSettings','struct','AcceptanceMask','int32','ArbitrationField','int32','TLCFileName','char')  RTIBlockParaDefault="struct('BoardTypeNo',4302,'BoardNo',1,'ChannelNo',1,'AcceptanceMask',0,'ArbitrationField',0,'Parameters',struct('Config',struct('Baudrate',500,'SampleMode',1,'UsedParamSet',1,'validSettings',1,'isBTRvalues',0,'Advanced',struct('Frequency',16000000,'BTR0',64,'BTR1',28,'Settings',struct('SMPL',0,'BRP',0,'NBT',16,'TSEG1',12,'TSEG2',1,'SJW',1,'SP',87))),'configType',1,'Options',struct('DataFileSelected',0,'DataFileName',{{['<no datafile support>']}},'DataFileDate',{{''}},'InterfaceFcn','rtican_dbc_file_parser','InterfaceFcnFileName','','LabelConfigType','volatile','AcceptanceMaskSelected',0,'MsgDataType','AllwaysDouble','NumType','hex','MaskType','STD','AcceptanceMask',0,'ArbitrationField',0,'UseMultipleMessageAccess',0),'RxReceiveStdOptions',struct('RxServiceStdEnabled',0,'RxServiceStdMsgIdent',1000,'RxServiceStdIdentNumType',1,'RxServiceStdIdentMask',0,'RxServiceStdMaskNumType',1,'RxServiceStdQueueSize',64),'RxReceiveXtdOptions',struct('RxServiceXtdEnabled',0,'RxServiceXtdMsgIdent',1001,'RxServiceXtdIdentNumType',1,'RxServiceXtdIdentMask',0,'RxServiceXtdMaskNumType',1,'RxServiceXtdQueueSize',64),'PartialNetworkingOptions',struct('switchedon',0,'format',1,'idmask',['    XXXXX XXXXXXXX XXXXXXXX XXXXXXXX'],'idcode','0','idfilter','0','datamaskused',0,'datalength',1,'datamask','0x0000000000000000','partialnetworkenable',0),'general',struct('Termination_common',1,'Termination_C252',1,'BusConfigurationRegister',0,'Transceiver','ISO11898','isFromLib',1)),'CCPParameters',struct('CRO',struct('Format','STD','NumFormat','hex','Id',1639),'DTO',struct('Format','STD','NumFormat','hex','Id',2017),'StationAdr',struct('NumFormat','hex','Value',57),'StationId',struct('Value',['dSPACE CCP Service']),'Enabled',0),'XCPParameters',struct('MASTER',struct('Format','STD','NumFormat','hex','Id',256),'SLAVE',struct('Format','STD','NumFormat','hex','Id',510),'Enabled',0,'PIDTransmissionEnabled',0),'GroupId',struct('Group',{{'RTICAN'}},'No',1,'Behavior',{{'EVER'}},'BlockType',{{'SOURCE'}},'NameChangeFlag',1),'SFcnRTICANSettings',struct('Baudrate',500,'configType',1,'AdvandedConfig',struct('Frequency',16000000,'BTR0','0x40','BTR1','0x1C'),'UsedParamSet',1,'STDMaskSelected','no','XTDMaskSelected','no','BoardType','DS4302','BoardNo',1,'ControllerNo',1,'Transceiver','ISO11898','BusConfigRegister',0,'TerminationRes',120,'UseMultipleMessageAccess','no','STDRXSrvcUsed','no','STDRXSrvcMsgId',1000,'STDRXSrvcMsgMask',0,'STDRXSrvcQueueSize',64,'XTDRXSrvcUsed','no','XTDRXSrvcMsgId',1001,'XTDRXSrvcQueueSize',64,'XTDRXSrvcMsgMask',0),'SFcnRTICCPSettings',struct('CRO',struct('Format','STD','NumFormat','hex','Id',1639),'DTO',struct('Format','STD','NumFormat','hex','Id',2017),'StationAdr',struct('NumFormat','hex','Value',57),'StationId',struct('Value',['dSPACE CCP Service']),'Enabled',0),'SFcnRTIXCPSettings',struct('MASTER',struct('Format','STD','NumFormat','hex','Id',256),'SLAVE',struct('Format','STD','NumFormat','hex','Id',510),'Enabled',0,'PIDTransmissionEnabled',0),'TLCFileName','rtican_master_setup')"
      settings: AttributesFormatString=Group Id: RTICAN3\n  SourceProductName=dSPACE RTI CAN Blockset
  CAN3 Status : rtican/RTICAN Status   Reserved1=[]  Reserved2=[]  Reserved3=[]  Reserved4=[]  DialogFcn=[]  UnitName=[]  SFcnRTICANStatus=[]  BoardTypeNo=[]  BoardNo=[]  ChannelNo=[]  Parameters=[]  Revision=[]  UnitValues=[]  DSProperties=struct('RTI',struct('Version',uint32(4),'BlockType',struct('isSLSource',uint8(1),'isSLSink',uint8(0),'isHWSource',uint8(0),'isHWSink',uint8(0),'isSetup',uint8(0),'isInline',uint8(1),'isNonInline',uint8(0),'isInterrupt',uint8(0),'isChannelwise',uint8(0)),'IOBoardType','RTICAN','UnitType','NON_MESSAGE','Identifier','STATUS','DialogType','ML','BlockSet','RTICAN','SlaveProcessor','CAN'))  RTIBlockInterface=struct('OutputPortsWidth',int32([1 1 1 1 1 1 1 1 1 1 1 1]),'OutputPortsActive',[1 1 1 1 1 1 1 1 1 1 0 0],'OutputPortsName',{{'Status',['Stuff errors'],['Format errors'],['Ack errors'],['Bit 0 errors'],['Bit 1 errors'],['CRC errors'],['RX lost'],['RX ok'],['TX ok'],['FT Status'],['FT error count']}},'OutputPortsDataType',{{'SS_UINT32','SS_UINT32','SS_UINT32','SS_UINT32','SS_UINT32','SS_UINT32','SS_UINT32','SS_UINT32','SS_UINT32','SS_UINT32','SS_UINT32','SS_UINT32'}},'DialogFcn','rtican_status_gui','BlockDisplay',{{'','center'}},'IconTransparency','on','ParameterTunableNames',{{}},'InitLevel',3,'BlockName',struct('Token',{{'CAN_TYPE','_STATUS_M','_C'}},'BlockParam',{{'BoardTypeNo','BoardNo','ChannelNo'}}),'SampleTime',{{2^-1}})  RTIBlockParameters=struct('BoardTypeNo',{{1,'OFF',[]}},'BoardNo',{{1,'ON',[1 16]}},'ChannelNo',{{2,'ON',[1 2]}},'Parameters',{{struct('general',struct('isFromLib',0,'StatusFlags',{{1;1;1;1;1;1;1;1;1;1;0;0}}),'options',struct('SampleTime',2^-1)),'OFF',[]}},'GroupId',{{struct('Group','RTICAN','No',3,'Behavior','NAMECHANGE','BlockType','SINK','NameChangeFlag',0),'OFF',[]}},'SFcnRTICANStatus',{{struct('Output',struct('Name',{'Status','StuffErrors','FormatErrors','AckErrors','Bit0Errors','Bit1Errors','CRCErrors','RXLost','RXOK','TXOK','FTStatus','FTErrorCount'},'Selected',{'yes','yes','yes','yes','yes','yes','yes','yes','yes','yes','no','no'}),'ControllerNo',2,'BoardNo',1,'BoardType','DS1','PortDatatype','UInt32'),'OFF',[]}},'TLCFileName',{{'rtican_status','OFF',[]}})  RTISFcnParameters=struct('SFcnRTICANStatus','struct','TLCFileName','char')  RTIBlockParaDefault=struct('BoardTypeNo',4302,'BoardNo',1,'ChannelNo',1,'Parameters',struct('general',struct('StatusFlags',{{1;1;1;1;1;1;1;1;1;1;0;0}},'isFromLib',1),'options',struct('SampleTime',2^-1)),'GroupId',struct('Group',{{'RTICAN'}},'No',1,'Behavior',{{'NAMECHANGE'}},'BlockType',{{'SINK'}},'NameChangeFlag',0),'SFcnRTICANStatus',struct('Output',struct('Name',{'Status','StuffErrors','FormatErrors','AckErrors','Bit0Errors','Bit1Errors','CRCErrors','RXLost','RXOK','TXOK','FTStatus','FTErrorCount'},'Selected',{'yes','yes','yes','yes','yes','yes','yes','yes','yes','yes','no','no'}),'ControllerNo',1,'BoardNo',1,'BoardType','DS4302','PortDatatype','real_T'),'TLCFileName','rtican_status')
      settings: AttributesFormatString=Group Id: RTICAN3\n  SourceProductName=dSPACE RTI CAN Blockset
  CAN_TYPE1_BOR_M2_C1 : rtican/RTICAN Bus Off Recovery   Reserved1=[]  Reserved2=[]  Reserved3=[]  Reserved4=[]  SfcnRTICANBusOff=[]  DialogFcn=[]  BoardTypeNo=[]  BoardNo=[]  ChannelNo=[]  Parameters=[]  UnitName=[]  Revision=[]  UnitValues=[]  DSProperties=struct('RTI',struct('Version',uint32(3),'BlockType',struct('isSLSource',uint8(0),'isSLSink',uint8(1),'isHWSource',uint8(1),'isHWSink',uint8(0),'isSetup',uint8(0),'isInline',uint8(1),'isNonInline',uint8(0),'isInterrupt',uint8(0),'isChannelwise',uint8(0)),'IOBoardType','RTICAN','UnitType','NON_MESSAGE','Identifier','BUS_OFF_RECOVERY','DialogType','ML','BlockSet','RTICAN','SlaveProcessor','CAN'))  RTIBlockInterface=struct('DialogFcn','rtican_bus_off_recovery_gui','BlockDisplay',{{['\nCAN\n Bus Off Recovery'],'center'}},'TriggerPort',{{'rising'}},'OutputPortsWidth',int32(0),'OutputPortsActive',0,'IconTransparency','on','InitLevel',3,'BlockName',struct('Token',{{'CAN_TYPE','_BOR_M','_C'}},'BlockParam',{{'BoardTypeNo','BoardNo','ChannelNo'}}))  RTIBlockParameters=struct('BoardTypeNo',{{1,'OFF',[]}},'BoardNo',{{2,'ON',[1 16]}},'ChannelNo',{{1,'ON',[1 2]}},'Parameters',{{struct('general',struct('isFromLib',0),'options',struct('TriggerType','rising')),'OFF',[]}},'GroupId',{{struct('Group',{{'RTICAN'}},'No',1,'Behavior',{{'NAMECHANGE'}},'BlockType',{{'SINK'}},'NameChangeFlag',0),'OFF',[]}},'SFcnRTICANBusOff',{{0,'OFF',[]}},'TLCFileName',{{'rtican_bus_off_recovery','OFF',[]}})  RTISFcnParameters=struct('SFcnRTICANBusOff','struct','TLCFileName','char')  RTIBlockParaDefault=struct('BoardTypeNo',4302,'BoardNo',1,'ChannelNo',1,'Parameters',struct('general',struct('isFromLib',1),'options',struct('TriggerType','rising')),'GroupId',struct('Group',{{'RTICAN'}},'No',1,'Behavior',{{'NAMECHANGE'}},'BlockType',{{'SINK'}},'NameChangeFlag',0),'SFcnRTICANBusOff',0,'TLCFileName','rtican_bus_off_recovery')
      settings: AttributesFormatString=Group Id: RTICAN1\n  SourceProductName=dSPACE RTI CAN Blockset
  USB_FLIGHT_REC_SETUP : rtiusbflightreclib/USB_FLIGHT_REC_SETUP  BufferOverwriteMode=Discard new data  TLCFileName=rtiusbflightrecsetup  DSProperties=struct('RTI',struct('Version',uint32(1),'BlockType',struct('isSLSource',uint8(0),'isSLSink',uint8(0),'isHWSource',uint8(0),'isHWSink',uint8(0),'isSetup',uint8(1),'isInline',uint8(1),'isNonInline',uint8(0),'isInterrupt',uint8(0),'isChannelwise',uint8(0)),'IOBoardType',{{'DSUSB','FLIGHTREC'}},'UnitType','FLIGHTREC','Identifier','SETUP','DialogType','SL','BlockSet','RTIUSBFLIGHTREC','SlaveProcessor','NONE'))  RTIBlockInterface=struct('OutputPortsActive',0,'OutputPortsWidth',int32(1),'BlockDisplay',{{['USB Flight Recorder\n Setup'],'center'}},'IconTransparency','off','InitLevel',3,'BlockName',struct('Token',{{'USB_FLIGHT_REC_SETUP'}}),'MaskDescription',['Initializes the USB device for flight recording.'])  RTIBlockParameters=struct('BufferOverwriteMode',{{1,'OFF',[1 2]}},'TLCFileName',{{'rtiusbflightrecsetup','OFF',[]}})  RTISFcnParameters=struct('BufferOverwriteMode','double','TLCFileName','char')  RTIBlockParaDefault=struct('BufferOverwriteMode',1,'TLCFileName','rtiusbflightrecsetup')
      settings: SourceProductName=dSPACE RTI USB Flight Rec Blockset
  wires:
  CAN 1 Recovery/1 -> CAN_TYPE1_BOR_M2_C1/Trigger

== system DR18E_Testpult/RTI Data ==
  RTI Data Store : Subsystem  Tag="struct('private',struct('version',struct('dsVer',uint32(2)),'access',struct('modified',['24-Feb-2019 16:37:57'],'type','Model','isPerm',1)),'public',struct('main',struct('data',[]),'sub',struct('name',{{'DR18E_Testpult'}},'data',{{struct('TH',struct('thTaskInfo',struct('taskType',{'TIMER','HWINT','TMRINT','SWINT','GLINT'},'tasksNumOf',{1,0,0,0,0},'srcIds',{{'TIMERA'},{},{},{},{}},'taskNames',{{['Timer Task 1']},{},{},{},{}})),'th_tc',struct('dataType','TASK','taskGroupId','','taskGroupList',{{}},'taskSchedulingPolicy','FCFS','taskType','TIMER','blkh',-1,'srcId','TIMERA','srcSgnName',['Timer A interrupt'],'srcCpuName','','taskName',['Timer Task 1  [0.001] s'],'taskNameDisplayExt','','smplTime',0.001,'smplTimeOffs',0,'hasFixedPriority',0,'priority',1,'hasFixedOvc',0,'ovcType',1,'ovcMax',1),'tc_th',struct('dataType','TASK','taskGroupId','','taskGroupList',{{}},'taskSchedulingPolicy','FCFS','taskType','TIMER','blkh',-1,'srcId','TIMERA','srcSgnName',['Timer A interrupt'],'srcCpuName','','taskName',['Timer Task 1  [0.001] s'],'taskNameDisplayExt','','smplTime',0.001,'smplTimeOffs',0,'hasFixedPriority',0,'priority',1,'hasFixedOvc',0,'ovcType',1,'ovcMax',1))}})))"  mask(RTI_DATA_STORE){}
      mask help:
      | RTI Data Store Block. This block is used by RTI to store internal model dependent data. Deleting this block will result in data loss.
      |
      | NEVER DELETE, COPY, OR MODIFY THIS BLOCK!
      mask Help:
      | RTI Data Store Block. This block is used by RTI to store internal model dependent data. Deleting this block will result in data loss.
      | 
      | NEVER DELETE, COPY, OR MODIFY THIS BLOCK!
      mask Display: text(0.5, 0.5, ' ', 'HorizontalAlignment', 'center');
